simulink model "ProximitySensor_Module"  (R2026a)
settings: Solver=VariableStepAuto
undefined symbols (not defined in the file): Sensor_FarRange_m, Sensor_NearRange_m
settings Model: Creator=ASUS  LastModifiedBy=ASUS

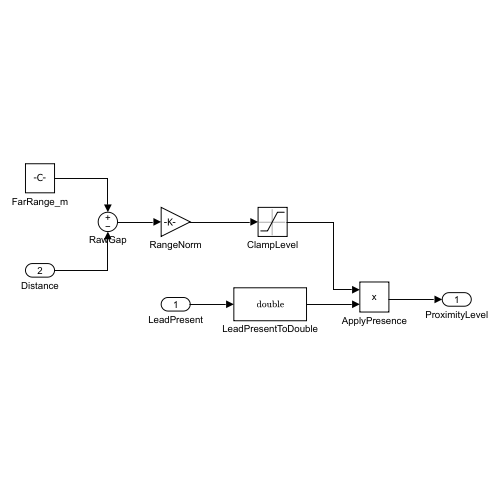
[thumbnail: Simulink's stored preview of the top-level diagram]
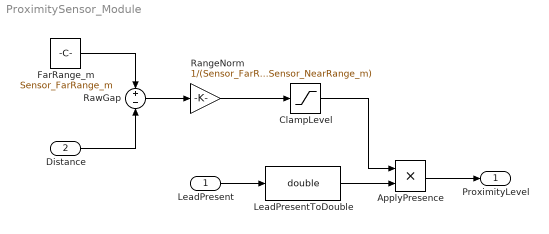
== system ProximitySensor_Module ==
  LeadPresent : Inport  OutDataTypeStr=boolean
  Distance : Inport  Port=2
  ApplyPresence : Product
  ClampLevel : Saturate  UpperLimit=1  LowerLimit=0
  FarRange_m : Constant  Value=Sensor_FarRange_m
  LeadPresentToDouble : DataTypeConversion  OutDataTypeStr=double
  RangeNorm : Gain  Gain=1/(Sensor_FarRange_m - Sensor_NearRange_m)
  RawGap : Sum  Inputs=+-
  ProximityLevel : Outport
  wires:
  ApplyPresence/1 -> ProximityLevel/1
  LeadPresentToDouble/1 -> ApplyPresence/2
  ClampLevel/1 -> ApplyPresence/1
  RangeNorm/1 -> ClampLevel/1
  RawGap/1 -> RangeNorm/1
  Distance/1 -> RawGap/2
  FarRange_m/1 -> RawGap/1
  LeadPresent/1 -> LeadPresentToDouble/1
